simulink model "cell_model_final2"  (R2023a)
settings: Solver=VariableStepAuto  StartTime=0.0  StopTime=T_e  RelTol=1e-3
libraries: neural x50, fl_lib x11, nesl_utility x11, BatteryEstimators x1, ee_lib x1, spspowerguiLib x1
(part 2 of 2)

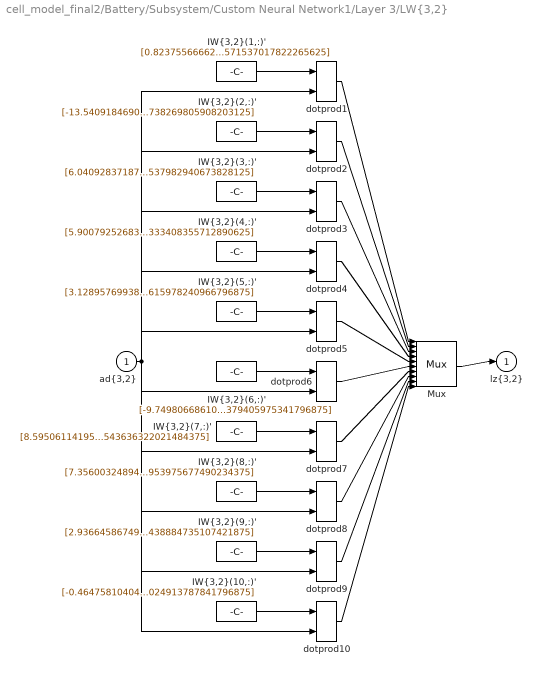
== system cell_model_final2/Battery/Subsystem/Custom Neural Network1/Layer 3/LW{3,2} ==
  "ad{3,2}" : Inport  PortDimensions=10
      mask Display: e = 0.06;c1 = [120 230 180]/255;c2 = ([120 230 180]+0)/(256+128);c3 = ([120 230 180]+128)/(256+128);patch([0 1 1 0],[0 0 1 1],c1);patch([0 1 1 1-e 1-e 0+e],[0 0 1 1-e 0+e 0+e],c2);patch([0 0 1 1-e 0+e 0+e],[0 1 1 1-e 1-e 0+e],c3);plot([0 1 1 0 0],[0 0 1 1 0]);
  "IW{3,2}(1,:)'" : Constant  Value=[0.8237556666211525158161066428874619305133819580078125;0.51571976457906709701006775503628887236118316650390625;-1.72538259025572227045586259919218719005584716796875;5.17857256433064350176209700293838977813720703125;-1.1681412187577204786492757193627767264842987060546875;1.1316882761782769417635563513613305985927581787109375;0.0112615445436738924323005761607419117353856563568115234375;-3.650864637324606309931596115347929298877716064453125;4.0848047341033453250247475807555019855499267578125;-3.444626401094726730889306054450571537017822265625]
      mask Display: e = 0.06;c1 = [120 150 230]/255;c2 = ([120 150 230]+0)/383;c3 = ([120 150 230]+128)/383;patch([0 1 1 0],[0 0 1 1],c1);patch([0 1 1 1-e 1-e 0+e],[0 0 1 1-e 0+e 0+e],c2);patch([0 0 1 1-e 0+e 0+e],[0 1 1 1-e 1-e 0+e],c3);plot([0 1 1 0 0],[0 0 1 1 0]);disp('weights');
  "IW{3,2}(10,:)'" : Constant  Value=[-0.464758104043701714136460623194579966366291046142578125;-0.5992515146409294057860961402184329926967620849609375;-0.251602361335951762999485481486772187054157257080078125;0.6197646560946881155729215606697835028171539306640625;-1.72620687903957392705933671095408499240875244140625;-0.367220886577844185527652598466374911367893218994140625;0.262110630021804624778525294459541328251361846923828125;-16.09438852063943414805180509574711322784423828125;-3.647089595181814303259670850820839405059814453125;-0.442257307555951495459112265962176024913787841796875]
      mask Display: e = 0.06;c1 = [120 150 230]/255;c2 = ([120 150 230]+0)/383;c3 = ([120 150 230]+128)/383;patch([0 1 1 0],[0 0 1 1],c1);patch([0 1 1 1-e 1-e 0+e],[0 0 1 1-e 0+e 0+e],c2);patch([0 0 1 1-e 0+e 0+e],[0 1 1 1-e 1-e 0+e],c3);plot([0 1 1 0 0],[0 0 1 1 0]);disp('weights');
  "IW{3,2}(2,:)'" : Constant  Value=[-13.54091846902824869403048069216310977935791015625;-7.78018168856120784226959585794247686862945556640625;-0.60416965064185490508208431492676027119159698486328125;11.427090964861445598899081232957541942596435546875;-8.1268851032437918746609284426085650920867919921875;2.555711316461996229776332256733439862728118896484375;-6.94223281636129652127920053317211568355560302734375;-3.618245010412151518863765886635519564151763916015625;-2.7533860611985634392340216436423361301422119140625;3.017057444568547186491969114285893738269805908203125]
      mask Display: e = 0.06;c1 = [120 150 230]/255;c2 = ([120 150 230]+0)/383;c3 = ([120 150 230]+128)/383;patch([0 1 1 0],[0 0 1 1],c1);patch([0 1 1 1-e 1-e 0+e],[0 0 1 1-e 0+e 0+e],c2);patch([0 0 1 1-e 0+e 0+e],[0 1 1 1-e 1-e 0+e],c3);plot([0 1 1 0 0],[0 0 1 1 0]);disp('weights');
  "IW{3,2}(3,:)'" : Constant  Value=[6.04092837187769848839025144116021692752838134765625;0.3393572733070511215913711566827259957790374755859375;-0.1361478471900444409126151867894805036485195159912109375;-0.61462706919321596910066318741883151233196258544921875;-1.7451047526482843519346488392329774796962738037109375;-0.8304746157176092768992248238646425306797027587890625;1.5984951728814287275071137628401629626750946044921875;-1.273854906771078265848018418182618916034698486328125;-0.57693518319445968867142937597236596047878265380859375;-1.594857872860516057045288107474334537982940673828125]
      mask Display: e = 0.06;c1 = [120 150 230]/255;c2 = ([120 150 230]+0)/383;c3 = ([120 150 230]+128)/383;patch([0 1 1 0],[0 0 1 1],c1);patch([0 1 1 1-e 1-e 0+e],[0 0 1 1-e 0+e 0+e],c2);patch([0 0 1 1-e 0+e 0+e],[0 1 1 1-e 1-e 0+e],c3);plot([0 1 1 0 0],[0 0 1 1 0]);disp('weights');
  "IW{3,2}(4,:)'" : Constant  Value=[5.9007925268365344351195744820870459079742431640625;-0.65084428298054064487843106689979322254657745361328125;2.17547306835202736152723446139134466648101806640625;-0.97304976004262166977554215918644331395626068115234375;0.23629131647569712182388457222259603440761566162109375;-0.7045430957878242583802830267813988029956817626953125;1.70831633299809926285206529428251087665557861328125;0.2704609371481063728737126439227722585201263427734375;-3.4953864206789848623202487942762672901153564453125;-0.6311199027205882661206715056323446333408355712890625]
      mask Display: e = 0.06;c1 = [120 150 230]/255;c2 = ([120 150 230]+0)/383;c3 = ([120 150 230]+128)/383;patch([0 1 1 0],[0 0 1 1],c1);patch([0 1 1 1-e 1-e 0+e],[0 0 1 1-e 0+e 0+e],c2);patch([0 0 1 1-e 0+e 0+e],[0 1 1 1-e 1-e 0+e],c3);plot([0 1 1 0 0],[0 0 1 1 0]);disp('weights');
  "IW{3,2}(5,:)'" : Constant  Value=[3.128957699389872004758217372000217437744140625;1.075965775142953884113694584812037646770477294921875;0.82378109590055481614712107329978607594966888427734375;-0.6107402140989381944535807633656077086925506591796875;-0.53224852174734793575083813266246579587459564208984375;0.501830234512349537823183709406293928623199462890625;0.11040997298376568902522620874151471070945262908935546875;-0.1498203391362867564762240135678439401090145111083984375;-0.2381298736799780935147197169499122537672519683837890625;-0.653770362514666469877511190134100615978240966796875]
      mask Display: e = 0.06;c1 = [120 150 230]/255;c2 = ([120 150 230]+0)/383;c3 = ([120 150 230]+128)/383;patch([0 1 1 0],[0 0 1 1],c1);patch([0 1 1 1-e 1-e 0+e],[0 0 1 1-e 0+e 0+e],c2);patch([0 0 1 1-e 0+e 0+e],[0 1 1 1-e 1-e 0+e],c3);plot([0 1 1 0 0],[0 0 1 1 0]);disp('weights');
  "IW{3,2}(6,:)'" : Constant  Value=[-9.74980668610820799813154735602438449859619140625;-6.3369232781815441057915450073778629302978515625;6.09327940852977345542740295059047639369964599609375;-4.7027926575543066434192951419390738010406494140625;-5.93152314487222209749006651691161096096038818359375;-15.5812875339934269192099236533977091312408447265625;-0.50925822907497264591114571885555051267147064208984375;2.883830636579010953113311188644729554653167724609375;4.20779319338805724015628584311343729496002197265625;0.10599562508165287499917184277364867739379405975341796875]
      mask Display: e = 0.06;c1 = [120 150 230]/255;c2 = ([120 150 230]+0)/383;c3 = ([120 150 230]+128)/383;patch([0 1 1 0],[0 0 1 1],c1);patch([0 1 1 1-e 1-e 0+e],[0 0 1 1-e 0+e 0+e],c2);patch([0 0 1 1-e 0+e 0+e],[0 1 1 1-e 1-e 0+e],c3);plot([0 1 1 0 0],[0 0 1 1 0]);disp('weights');
  "IW{3,2}(7,:)'" : Constant  Value=[8.5950611419544902247480422374792397022247314453125;1.5635822242984642738150569130084477365016937255859375;3.771727767111268558863912403467111289501190185546875;-1.0919709536841548658259171133977361023426055908203125;11.791071227848863856024763663299381732940673828125;1.6213272379689993574203299431246705353260040283203125;1.5352528648102532482511151101789437234401702880859375;15.361914640598907766388947493396699428558349609375;-11.2104874541272163668281791615299880504608154296875;-19.9152018216922215287922881543636322021484375]
      mask Display: e = 0.06;c1 = [120 150 230]/255;c2 = ([120 150 230]+0)/383;c3 = ([120 150 230]+128)/383;patch([0 1 1 0],[0 0 1 1],c1);patch([0 1 1 1-e 1-e 0+e],[0 0 1 1-e 0+e 0+e],c2);patch([0 0 1 1-e 0+e 0+e],[0 1 1 1-e 1-e 0+e],c3);plot([0 1 1 0 0],[0 0 1 1 0]);disp('weights');
  "IW{3,2}(8,:)'" : Constant  Value=[7.35600324894948442988606984727084636688232421875;0.77271926047475936183417388747329823672771453857421875;0.464109698369803924666854300085105933248996734619140625;0.79881594776103026500635451156995259225368499755859375;-1.193220098882364244019527177442796528339385986328125;-1.7205400623213764621510790675529278814792633056640625;1.884626601101445420027857835520990192890167236328125;-0.85140840144191176630528161695110611617565155029296875;3.348620010332649332696064448100514709949493408203125;0.518919361702509629452606532140634953975677490234375]
      mask Display: e = 0.06;c1 = [120 150 230]/255;c2 = ([120 150 230]+0)/383;c3 = ([120 150 230]+128)/383;patch([0 1 1 0],[0 0 1 1],c1);patch([0 1 1 1-e 1-e 0+e],[0 0 1 1-e 0+e 0+e],c2);patch([0 0 1 1-e 0+e 0+e],[0 1 1 1-e 1-e 0+e],c3);plot([0 1 1 0 0],[0 0 1 1 0]);disp('weights');
  "IW{3,2}(9,:)'" : Constant  Value=[2.9366458674975319809163920581340789794921875;0.11382377123805066665429563954603509046137332916259765625;-0.180298572854895533534858031998737715184688568115234375;-1.4519372197763338316889303314383141696453094482421875;2.490459681232118693827715105726383626461029052734375;-1.0414472033151138674611502210609614849090576171875;-3.008464300367092558730064411065541207790374755859375;1.7983374122680337858781740578706376254558563232421875;-0.14493642436333631362543883369653485715389251708984375;0.08730435018556663429034614409829373471438884735107421875]
      mask Display: e = 0.06;c1 = [120 150 230]/255;c2 = ([120 150 230]+0)/383;c3 = ([120 150 230]+128)/383;patch([0 1 1 0],[0 0 1 1],c1);patch([0 1 1 1-e 1-e 0+e],[0 0 1 1-e 0+e 0+e],c2);patch([0 0 1 1-e 0+e 0+e],[0 1 1 1-e 1-e 0+e],c3);plot([0 1 1 0 0],[0 0 1 1 0]);disp('weights');
  Mux : Mux  Inputs=10
      mask Display: e = 0.06;c1 = [120 150 230]/255;c2 = ([120 150 230]+0)/383;c3 = ([120 150 230]+128)/383;patch([0 1 1 0],[0 0 1 1],c1);patch([0 1 1 1-e 1-e 0+e],[0 0 1 1-e 0+e 0+e],c2);patch([0 0 1 1-e 0+e 0+e],[0 1 1 1-e 1-e 0+e],c3);plot([0 1 1 0 0],[0 0 1 1 0]);disp('Mux');
  dotprod{1..10} (10 alike) : neural/Weight Functions/dotprod
  "lz{3,2}" : Outport
      mask Display: e = 0.06;c1 = [120 230 180]/255;c2 = ([120 230 180]+0)/(256+128);c3 = ([120 230 180]+128)/(256+128);patch([0 1 1 0],[0 0 1 1],c1);patch([0 1 1 1-e 1-e 0+e],[0 0 1 1-e 0+e 0+e],c2);patch([0 0 1 1-e 0+e 0+e],[0 1 1 1-e 1-e 0+e],c3);plot([0 1 1 0 0],[0 0 1 1 0]);
  wires:
  "IW{3,2}(1,:)'"/1 -> dotprod1/1
  "ad{3,2}"/1 -> dotprod1/2, dotprod2/2, dotprod3/2, dotprod4/2, dotprod5/2, dotprod6/2, dotprod7/2, dotprod8/2, dotprod9/2, dotprod10/2
  dotprod1/1 -> Mux/1
  "IW{3,2}(2,:)'"/1 -> dotprod2/1
  dotprod2/1 -> Mux/2
  "IW{3,2}(3,:)'"/1 -> dotprod3/1
  dotprod3/1 -> Mux/3
  "IW{3,2}(4,:)'"/1 -> dotprod4/1
  dotprod4/1 -> Mux/4
  "IW{3,2}(5,:)'"/1 -> dotprod5/1
  dotprod5/1 -> Mux/5
  "IW{3,2}(6,:)'"/1 -> dotprod6/1
  dotprod6/1 -> Mux/6
  "IW{3,2}(7,:)'"/1 -> dotprod7/1
  dotprod7/1 -> Mux/7
  "IW{3,2}(8,:)'"/1 -> dotprod8/1
  dotprod8/1 -> Mux/8
  "IW{3,2}(9,:)'"/1 -> dotprod9/1
  dotprod9/1 -> Mux/9
  "IW{3,2}(10,:)'"/1 -> dotprod10/1
  dotprod10/1 -> Mux/10
  Mux/1 -> "lz{3,2}"/1

== system cell_model_final2/Battery/Subsystem/Custom Neural Network1/Layer 4/Delays 1 ==
  "p{4}" : Inport  PortDimensions=10
      mask Display: e = 0.06;c1 = [120 230 180]/255;c2 = ([120 230 180]+0)/(256+128);c3 = ([120 230 180]+128)/(256+128);patch([0 1 1 0],[0 0 1 1],c1);patch([0 1 1 1-e 1-e 0+e],[0 0 1 1-e 0+e 0+e],c2);patch([0 0 1 1-e 0+e 0+e],[0 1 1 1-e 1-e 0+e],c3);plot([0 1 1 0 0],[0 0 1 1 0]);
  mux : Mux  Inputs=1
      mask Display: e = 0.06;c1 = [120 150 230]/255;c2 = ([120 150 230]+0)/383;c3 = ([120 150 230]+128)/383;patch([0 1 1 0],[0 0 1 1],c1);patch([0 1 1 1-e 1-e 0+e],[0 0 1 1-e 0+e 0+e],c2);patch([0 0 1 1-e 0+e 0+e],[0 1 1 1-e 1-e 0+e],c3);plot([0 1 1 0 0],[0 0 1 1 0]);disp('Mux')
  "pd{4,3}" : Outport
      mask Display: e = 0.06;c1 = [120 230 180]/255;c2 = ([120 230 180]+0)/(256+128);c3 = ([120 230 180]+128)/(256+128);patch([0 1 1 0],[0 0 1 1],c1);patch([0 1 1 1-e 1-e 0+e],[0 0 1 1-e 0+e 0+e],c2);patch([0 0 1 1-e 0+e 0+e],[0 1 1 1-e 1-e 0+e],c3);plot([0 1 1 0 0],[0 0 1 1 0]);
  wires:
  "p{4}"/1 -> mux/1
  mux/1 -> "pd{4,3}"/1

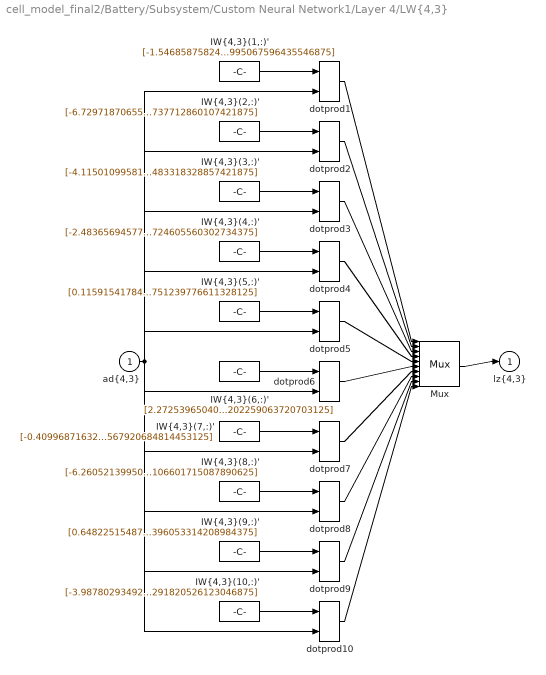
== system cell_model_final2/Battery/Subsystem/Custom Neural Network1/Layer 4/LW{4,3} ==
  "ad{4,3}" : Inport  PortDimensions=10
      mask Display: e = 0.06;c1 = [120 230 180]/255;c2 = ([120 230 180]+0)/(256+128);c3 = ([120 230 180]+128)/(256+128);patch([0 1 1 0],[0 0 1 1],c1);patch([0 1 1 1-e 1-e 0+e],[0 0 1 1-e 0+e 0+e],c2);patch([0 0 1 1-e 0+e 0+e],[0 1 1 1-e 1-e 0+e],c3);plot([0 1 1 0 0],[0 0 1 1 0]);
  "IW{4,3}(1,:)'" : Constant  Value=[-1.546858758243345288718728625099174678325653076171875;-5.41574496058701715384131603059358894824981689453125;-3.346839046542495754721358025562949478626251220703125;0.451767824527080197327677524299360811710357666015625;-6.669883365719584844555356539785861968994140625;-0.62066255443102724687065574471489526331424713134765625;-1.96645724734477322925840780953876674175262451171875;1.31646724517947699695241681183688342571258544921875;-5.08626513682391223625245402217842638492584228515625;0.6517186992629386832476257040980271995067596435546875]
      mask Display: e = 0.06;c1 = [120 150 230]/255;c2 = ([120 150 230]+0)/383;c3 = ([120 150 230]+128)/383;patch([0 1 1 0],[0 0 1 1],c1);patch([0 1 1 1-e 1-e 0+e],[0 0 1 1-e 0+e 0+e],c2);patch([0 0 1 1-e 0+e 0+e],[0 1 1 1-e 1-e 0+e],c3);plot([0 1 1 0 0],[0 0 1 1 0]);disp('weights');
  "IW{4,3}(10,:)'" : Constant  Value=[-3.98780293492059367821411797194741666316986083984375;3.26630480238409592885773236048407852649688720703125;-5.634060446159356416728769545443356037139892578125;1.3065505122799716541948100712033919990062713623046875;4.9805298971298146426534003694541752338409423828125;-6.1388756929773773407532644341699779033660888671875;-0.046357114954881643853479289418828557245433330535888671875;3.15372981633694760006392243667505681514739990234375;7.0811699029023547069527921848930418491363525390625;1.955086813922487731787214215728454291820526123046875]
      mask Display: e = 0.06;c1 = [120 150 230]/255;c2 = ([120 150 230]+0)/383;c3 = ([120 150 230]+128)/383;patch([0 1 1 0],[0 0 1 1],c1);patch([0 1 1 1-e 1-e 0+e],[0 0 1 1-e 0+e 0+e],c2);patch([0 0 1 1-e 0+e 0+e],[0 1 1 1-e 1-e 0+e],c3);plot([0 1 1 0 0],[0 0 1 1 0]);disp('weights');
  "IW{4,3}(2,:)'" : Constant  Value=[-6.72971870655333237465356432949192821979522705078125;1.7518616056329172625538603824679739773273468017578125;9.13726051001393813066897564567625522613525390625;-4.57532989411322699169204497593455016613006591796875;4.633243645744716587842049193568527698516845703125;3.275645115094608872396975129959173500537872314453125;1.1143148869915915355477409320883452892303466796875;-7.5247483965626695834316706168465316295623779296875;17.269833940598214638839635881595313549041748046875;-27.999460156409394784304822678677737712860107421875]
      mask Display: e = 0.06;c1 = [120 150 230]/255;c2 = ([120 150 230]+0)/383;c3 = ([120 150 230]+128)/383;patch([0 1 1 0],[0 0 1 1],c1);patch([0 1 1 1-e 1-e 0+e],[0 0 1 1-e 0+e 0+e],c2);patch([0 0 1 1-e 0+e 0+e],[0 1 1 1-e 1-e 0+e],c3);plot([0 1 1 0 0],[0 0 1 1 0]);disp('weights');
  "IW{4,3}(3,:)'" : Constant  Value=[-4.11501099581523011039507764508016407489776611328125;-0.81767388943092333963846840561018325388431549072265625;1.9110066220211112675286813100683502852916717529296875;-1.0348181098407638334180091987946070730686187744140625;-10.8015348074335815198310228879563510417938232421875;5.81950150578970948345158831216394901275634765625;5.04756186786198046689833063283003866672515869140625;-3.39679740951199082843459109426476061344146728515625;-8.4884899486503844201479296316392719745635986328125;-0.0916084538988721497343448163519497029483318328857421875]
      mask Display: e = 0.06;c1 = [120 150 230]/255;c2 = ([120 150 230]+0)/383;c3 = ([120 150 230]+128)/383;patch([0 1 1 0],[0 0 1 1],c1);patch([0 1 1 1-e 1-e 0+e],[0 0 1 1-e 0+e 0+e],c2);patch([0 0 1 1-e 0+e 0+e],[0 1 1 1-e 1-e 0+e],c3);plot([0 1 1 0 0],[0 0 1 1 0]);disp('weights');
  "IW{4,3}(4,:)'" : Constant  Value=[-2.483656945778097036026110799866728484630584716796875;0.7278102331529456847647452377714216709136962890625;2.740000688501283310216649624635465443134307861328125;-5.623990090066673275259745423682034015655517578125;-0.94208172703027648342555266935960389673709869384765625;1.2687902289863941529546309539000503718852996826171875;2.67200420830051132980997863342054188251495361328125;-2.153123444341618952790895491489209234714508056640625;4.57178011351702284770226469845511019229888916015625;-6.047806784650131106673143221996724605560302734375]
      mask Display: e = 0.06;c1 = [120 150 230]/255;c2 = ([120 150 230]+0)/383;c3 = ([120 150 230]+128)/383;patch([0 1 1 0],[0 0 1 1],c1);patch([0 1 1 1-e 1-e 0+e],[0 0 1 1-e 0+e 0+e],c2);patch([0 0 1 1-e 0+e 0+e],[0 1 1 1-e 1-e 0+e],c3);plot([0 1 1 0 0],[0 0 1 1 0]);disp('weights');
  "IW{4,3}(5,:)'" : Constant  Value=[0.1159154178461006823308565572006045840680599212646484375;-1.8499853959098986333486891453503631055355072021484375;1.2848704877071168706237358492217026650905609130859375;-2.157547822042106933082550312974490225315093994140625;-4.241359906210082186817089677788317203521728515625;0.57736464622362737575400615241960622370243072509765625;-0.01329290190106735027042450525414096773602068424224853515625;-0.74914529347293534744522958135348744690418243408203125;-0.06294257075587723904153136800232459791004657745361328125;-1.23916661798865135324376751668751239776611328125]
      mask Display: e = 0.06;c1 = [120 150 230]/255;c2 = ([120 150 230]+0)/383;c3 = ([120 150 230]+128)/383;patch([0 1 1 0],[0 0 1 1],c1);patch([0 1 1 1-e 1-e 0+e],[0 0 1 1-e 0+e 0+e],c2);patch([0 0 1 1-e 0+e 0+e],[0 1 1 1-e 1-e 0+e],c3);plot([0 1 1 0 0],[0 0 1 1 0]);disp('weights');
  "IW{4,3}(6,:)'" : Constant  Value=[2.2725396504043171574949155910871922969818115234375;1.73565961087123010742061524069868028163909912109375;-1.569911766278661247042691684328019618988037109375;3.30693627073573903629721826291643083095550537109375;0.05289787163614211029649680995134986005723476409912109375;-8.7957836952562242771591627388261258602142333984375;2.29184513753000640434720480698160827159881591796875;-2.832488029926452099971356801688671112060546875;0.7825427923264813845349863186129368841648101806640625;-3.85471441436257311607960218680091202259063720703125]
      mask Display: e = 0.06;c1 = [120 150 230]/255;c2 = ([120 150 230]+0)/383;c3 = ([120 150 230]+128)/383;patch([0 1 1 0],[0 0 1 1],c1);patch([0 1 1 1-e 1-e 0+e],[0 0 1 1-e 0+e 0+e],c2);patch([0 0 1 1-e 0+e 0+e],[0 1 1 1-e 1-e 0+e],c3);plot([0 1 1 0 0],[0 0 1 1 0]);disp('weights');
  "IW{4,3}(7,:)'" : Constant  Value=[-0.409968716321139903246972835404449142515659332275390625;-0.6642236348449463978482754100696183741092681884765625;2.4107726960936570748117446782998740673065185546875;3.3503577009520579821355568128637969493865966796875;-3.37791576775854185399339257855899631977081298828125;-4.03534815408382296908484931918792426586151123046875;0.88018778310807543885374570891144685447216033935546875;3.60491302059822782410947183961980044841766357421875;5.2728163588108483139649251825176179409027099609375;0.171802163157868836851349669814226217567920684814453125]
      mask Display: e = 0.06;c1 = [120 150 230]/255;c2 = ([120 150 230]+0)/383;c3 = ([120 150 230]+128)/383;patch([0 1 1 0],[0 0 1 1],c1);patch([0 1 1 1-e 1-e 0+e],[0 0 1 1-e 0+e 0+e],c2);patch([0 0 1 1-e 0+e 0+e],[0 1 1 1-e 1-e 0+e],c3);plot([0 1 1 0 0],[0 0 1 1 0]);disp('weights');
  "IW{4,3}(8,:)'" : Constant  Value=[-6.26052139950341679508483139215968549251556396484375;14.977608629465382961143404827453196048736572265625;-12.272214380771313102513886406086385250091552734375;13.1246927787515037522325656027533113956451416015625;-3.196246741237889654740911282715387642383575439453125;4.721382732960687889089967939071357250213623046875;0.90901296199383907481461619681795127689838409423828125;-4.89929433066750785741305662668310105800628662109375;14.120534296999966983321428415365517139434814453125;10.1202950796688586621030481182970106601715087890625]
      mask Display: e = 0.06;c1 = [120 150 230]/255;c2 = ([120 150 230]+0)/383;c3 = ([120 150 230]+128)/383;patch([0 1 1 0],[0 0 1 1],c1);patch([0 1 1 1-e 1-e 0+e],[0 0 1 1-e 0+e 0+e],c2);patch([0 0 1 1-e 0+e 0+e],[0 1 1 1-e 1-e 0+e],c3);plot([0 1 1 0 0],[0 0 1 1 0]);disp('weights');
  "IW{4,3}(9,:)'" : Constant  Value=[0.648225154879653597816968613187782466411590576171875;14.361668336610517116014307248406112194061279296875;2.986517236766482508159015196724794805049896240234375;-8.499556907750882572827322292141616344451904296875;14.8883666792993221150709359790198504924774169921875;11.4168531391206879987976208212785422801971435546875;-10.8986631467053118882404305622912943363189697265625;-15.0582136542635165454839807352982461452484130859375;-0.86265019356548078288682290803990326821804046630859375;-24.31247704679903876012758701108396053314208984375]
      mask Display: e = 0.06;c1 = [120 150 230]/255;c2 = ([120 150 230]+0)/383;c3 = ([120 150 230]+128)/383;patch([0 1 1 0],[0 0 1 1],c1);patch([0 1 1 1-e 1-e 0+e],[0 0 1 1-e 0+e 0+e],c2);patch([0 0 1 1-e 0+e 0+e],[0 1 1 1-e 1-e 0+e],c3);plot([0 1 1 0 0],[0 0 1 1 0]);disp('weights');
  Mux : Mux  Inputs=10
      mask Display: e = 0.06;c1 = [120 150 230]/255;c2 = ([120 150 230]+0)/383;c3 = ([120 150 230]+128)/383;patch([0 1 1 0],[0 0 1 1],c1);patch([0 1 1 1-e 1-e 0+e],[0 0 1 1-e 0+e 0+e],c2);patch([0 0 1 1-e 0+e 0+e],[0 1 1 1-e 1-e 0+e],c3);plot([0 1 1 0 0],[0 0 1 1 0]);disp('Mux');
  dotprod{1..10} (10 alike) : neural/Weight Functions/dotprod
  "lz{4,3}" : Outport
      mask Display: e = 0.06;c1 = [120 230 180]/255;c2 = ([120 230 180]+0)/(256+128);c3 = ([120 230 180]+128)/(256+128);patch([0 1 1 0],[0 0 1 1],c1);patch([0 1 1 1-e 1-e 0+e],[0 0 1 1-e 0+e 0+e],c2);patch([0 0 1 1-e 0+e 0+e],[0 1 1 1-e 1-e 0+e],c3);plot([0 1 1 0 0],[0 0 1 1 0]);
  wires:
  "IW{4,3}(1,:)'"/1 -> dotprod1/1
  "ad{4,3}"/1 -> dotprod1/2, dotprod2/2, dotprod3/2, dotprod4/2, dotprod5/2, dotprod6/2, dotprod7/2, dotprod8/2, dotprod9/2, dotprod10/2
  dotprod1/1 -> Mux/1
  "IW{4,3}(2,:)'"/1 -> dotprod2/1
  dotprod2/1 -> Mux/2
  "IW{4,3}(3,:)'"/1 -> dotprod3/1
  dotprod3/1 -> Mux/3
  "IW{4,3}(4,:)'"/1 -> dotprod4/1
  dotprod4/1 -> Mux/4
  "IW{4,3}(5,:)'"/1 -> dotprod5/1
  dotprod5/1 -> Mux/5
  "IW{4,3}(6,:)'"/1 -> dotprod6/1
  dotprod6/1 -> Mux/6
  "IW{4,3}(7,:)'"/1 -> dotprod7/1
  dotprod7/1 -> Mux/7
  "IW{4,3}(8,:)'"/1 -> dotprod8/1
  dotprod8/1 -> Mux/8
  "IW{4,3}(9,:)'"/1 -> dotprod9/1
  dotprod9/1 -> Mux/9
  "IW{4,3}(10,:)'"/1 -> dotprod10/1
  dotprod10/1 -> Mux/10
  Mux/1 -> "lz{4,3}"/1

== system cell_model_final2/Battery/Subsystem/Custom Neural Network1/Layer 5/Delays 1 ==
  "p{5}" : Inport  PortDimensions=10
      mask Display: e = 0.06;c1 = [120 230 180]/255;c2 = ([120 230 180]+0)/(256+128);c3 = ([120 230 180]+128)/(256+128);patch([0 1 1 0],[0 0 1 1],c1);patch([0 1 1 1-e 1-e 0+e],[0 0 1 1-e 0+e 0+e],c2);patch([0 0 1 1-e 0+e 0+e],[0 1 1 1-e 1-e 0+e],c3);plot([0 1 1 0 0],[0 0 1 1 0]);
  mux : Mux  Inputs=1
      mask Display: e = 0.06;c1 = [120 150 230]/255;c2 = ([120 150 230]+0)/383;c3 = ([120 150 230]+128)/383;patch([0 1 1 0],[0 0 1 1],c1);patch([0 1 1 1-e 1-e 0+e],[0 0 1 1-e 0+e 0+e],c2);patch([0 0 1 1-e 0+e 0+e],[0 1 1 1-e 1-e 0+e],c3);plot([0 1 1 0 0],[0 0 1 1 0]);disp('Mux')
  "pd{5,4}" : Outport
      mask Display: e = 0.06;c1 = [120 230 180]/255;c2 = ([120 230 180]+0)/(256+128);c3 = ([120 230 180]+128)/(256+128);patch([0 1 1 0],[0 0 1 1],c1);patch([0 1 1 1-e 1-e 0+e],[0 0 1 1-e 0+e 0+e],c2);patch([0 0 1 1-e 0+e 0+e],[0 1 1 1-e 1-e 0+e],c3);plot([0 1 1 0 0],[0 0 1 1 0]);
  wires:
  "p{5}"/1 -> mux/1
  mux/1 -> "pd{5,4}"/1

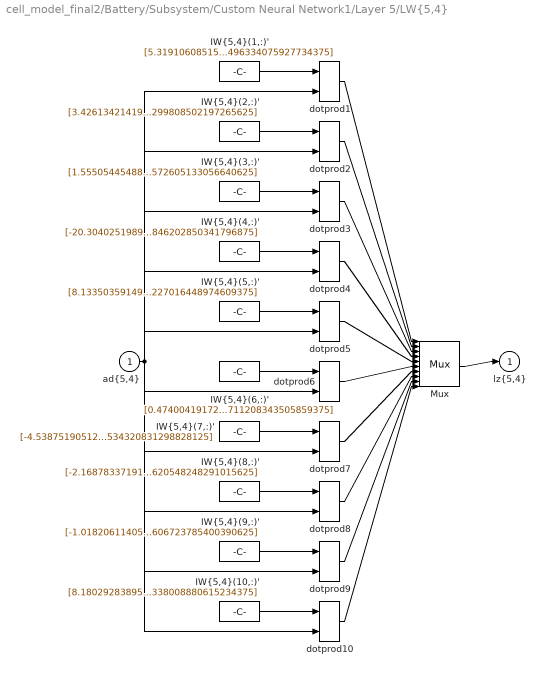
== system cell_model_final2/Battery/Subsystem/Custom Neural Network1/Layer 5/LW{5,4} ==
  "ad{5,4}" : Inport  PortDimensions=10
      mask Display: e = 0.06;c1 = [120 230 180]/255;c2 = ([120 230 180]+0)/(256+128);c3 = ([120 230 180]+128)/(256+128);patch([0 1 1 0],[0 0 1 1],c1);patch([0 1 1 1-e 1-e 0+e],[0 0 1 1-e 0+e 0+e],c2);patch([0 0 1 1-e 0+e 0+e],[0 1 1 1-e 1-e 0+e],c3);plot([0 1 1 0 0],[0 0 1 1 0]);
  "IW{5,4}(1,:)'" : Constant  Value=[5.31910608515874283597213434404693543910980224609375;-37.6187219247760680218561901710927486419677734375;-1.434327602098746989867095180670730769634246826171875;-1.3067931540625294939417244677315466105937957763671875;0.08338336636821926106666325040350784547626972198486328125;3.10444042714829127049824819550849497318267822265625;3.20260944459612328927278213086538016796112060546875;0.69515320195009311365907933577545918524265289306640625;1.22868083139611439236205114866606891155242919921875;-5.956084539158521096169351949356496334075927734375]
      mask Display: e = 0.06;c1 = [120 150 230]/255;c2 = ([120 150 230]+0)/383;c3 = ([120 150 230]+128)/383;patch([0 1 1 0],[0 0 1 1],c1);patch([0 1 1 1-e 1-e 0+e],[0 0 1 1-e 0+e 0+e],c2);patch([0 0 1 1-e 0+e 0+e],[0 1 1 1-e 1-e 0+e],c3);plot([0 1 1 0 0],[0 0 1 1 0]);disp('weights');
  "IW{5,4}(10,:)'" : Constant  Value=[8.18029283895581471597324707545340061187744140625;-0.86604032375827444401039656440843828022480010986328125;10.406226965972205533716987702064216136932373046875;-8.485710592220481629510686616413295269012451171875;-0.251726104378499015989945064575294964015483856201171875;20.0634977846928421740813064388930797576904296875;-1.366718568608316086709919545683078467845916748046875;27.82724288856896777133442810736596584320068359375;4.8484804648080181976865787873975932598114013671875;3.57714877656545038320246021612547338008880615234375]
      mask Display: e = 0.06;c1 = [120 150 230]/255;c2 = ([120 150 230]+0)/383;c3 = ([120 150 230]+128)/383;patch([0 1 1 0],[0 0 1 1],c1);patch([0 1 1 1-e 1-e 0+e],[0 0 1 1-e 0+e 0+e],c2);patch([0 0 1 1-e 0+e 0+e],[0 1 1 1-e 1-e 0+e],c3);plot([0 1 1 0 0],[0 0 1 1 0]);disp('weights');
  "IW{5,4}(2,:)'" : Constant  Value=[3.42613421419545005619511357508599758148193359375;1.114618823772122624404801172204315662384033203125;-6.75680619223893419444948449381627142429351806640625;-1.91855581646149797592215691111050546169281005859375;-3.572382975305118169018214757670648396015167236328125;4.45780515936019838818538119085133075714111328125;-5.79158021666007538641451901639811694622039794921875;4.38311052670753742432907529291696846485137939453125;-1.7471431694872290307785078766755759716033935546875;-1.199354747415134259114211090491153299808502197265625]
      mask Display: e = 0.06;c1 = [120 150 230]/255;c2 = ([120 150 230]+0)/383;c3 = ([120 150 230]+128)/383;patch([0 1 1 0],[0 0 1 1],c1);patch([0 1 1 1-e 1-e 0+e],[0 0 1 1-e 0+e 0+e],c2);patch([0 0 1 1-e 0+e 0+e],[0 1 1 1-e 1-e 0+e],c3);plot([0 1 1 0 0],[0 0 1 1 0]);disp('weights');
  "IW{5,4}(3,:)'" : Constant  Value=[1.555054454884164716332861644332297146320343017578125;0.280436030021297078018704951318795792758464813232421875;-1.340061650945262083922671081381849944591522216796875;1.6251508867869788321769419781048782169818878173828125;-1.0157386511680421836700816129450686275959014892578125;-5.35130459212175946248635227675549685955047607421875;0.76519595505605464413889649222255684435367584228515625;0.2585494067780447213777961223968304693698883056640625;0.7317476832289095955985658292775042355060577392578125;-1.637176688866903706554012387641705572605133056640625]
      mask Display: e = 0.06;c1 = [120 150 230]/255;c2 = ([120 150 230]+0)/383;c3 = ([120 150 230]+128)/383;patch([0 1 1 0],[0 0 1 1],c1);patch([0 1 1 1-e 1-e 0+e],[0 0 1 1-e 0+e 0+e],c2);patch([0 0 1 1-e 0+e 0+e],[0 1 1 1-e 1-e 0+e],c3);plot([0 1 1 0 0],[0 0 1 1 0]);disp('weights');
  "IW{5,4}(4,:)'" : Constant  Value=[-20.30402519890122903234441764652729034423828125;22.457629621246137929801989230327308177947998046875;0.314878492933852116575366153483628295361995697021484375;-44.36293643056806246249834657646715641021728515625;7.3827011574238969870975779485888779163360595703125;-35.88281999329792171238295850344002246856689453125;60.188644212525076682140934281051158905029296875;-8.9725237313902770353024607175029814243316650390625;-7.32605500412379928576456222799606621265411376953125;20.154382584722309701419362681917846202850341796875]
      mask Display: e = 0.06;c1 = [120 150 230]/255;c2 = ([120 150 230]+0)/383;c3 = ([120 150 230]+128)/383;patch([0 1 1 0],[0 0 1 1],c1);patch([0 1 1 1-e 1-e 0+e],[0 0 1 1-e 0+e 0+e],c2);patch([0 0 1 1-e 0+e 0+e],[0 1 1 1-e 1-e 0+e],c3);plot([0 1 1 0 0],[0 0 1 1 0]);disp('weights');
  "IW{5,4}(5,:)'" : Constant  Value=[8.1335035914949518343064482905901968479156494140625;15.49384820678261576176737435162067413330078125;37.736545982073863569894456304609775543212890625;-13.3628093022243650267455450375564396381378173828125;-8.62393036572091631342118489556014537811279296875;-16.40819498321757663461539777927100658416748046875;-3.410303327601974299199127926840446889400482177734375;24.133962885927786601314437575638294219970703125;-16.080026613818450442749963258393108844757080078125;9.37803262099551915298434323631227016448974609375]
      mask Display: e = 0.06;c1 = [120 150 230]/255;c2 = ([120 150 230]+0)/383;c3 = ([120 150 230]+128)/383;patch([0 1 1 0],[0 0 1 1],c1);patch([0 1 1 1-e 1-e 0+e],[0 0 1 1-e 0+e 0+e],c2);patch([0 0 1 1-e 0+e 0+e],[0 1 1 1-e 1-e 0+e],c3);plot([0 1 1 0 0],[0 0 1 1 0]);disp('weights');
  "IW{5,4}(6,:)'" : Constant  Value=[0.474004191724247625483457113659824244678020477294921875;-0.771879334027128383155513802194036543369293212890625;1.25980116172532152774010683060623705387115478515625;5.09481225898411604902094040880911052227020263671875;-6.057666156447250926930792047642171382904052734375;1.0032813129573601163002649627742357552051544189453125;0.54980960210650720032532490222365595400333404541015625;5.677288355257385177310425206087529659271240234375;3.371131008149129026918444651528261601924896240234375;0.339900525159732236346599165699444711208343505859375]
      mask Display: e = 0.06;c1 = [120 150 230]/255;c2 = ([120 150 230]+0)/383;c3 = ([120 150 230]+128)/383;patch([0 1 1 0],[0 0 1 1],c1);patch([0 1 1 1-e 1-e 0+e],[0 0 1 1-e 0+e 0+e],c2);patch([0 0 1 1-e 0+e 0+e],[0 1 1 1-e 1-e 0+e],c3);plot([0 1 1 0 0],[0 0 1 1 0]);disp('weights');
  "IW{5,4}(7,:)'" : Constant  Value=[-4.53875190512472048709469163441099226474761962890625;-1.27624362940507030117487374809570610523223876953125;-0.5325326436101438520864803649601526558399200439453125;-0.76454466657364406056984762471984140574932098388671875;1.3293898148616258847454218994244001805782318115234375;8.2016192404383243541587944491766393184661865234375;-0.420980338568227863138559996514231897890567779541015625;-0.32581960761651063140931228190311230719089508056640625;3.68923545619525139471761576714925467967987060546875;3.654730298709310876148492752690799534320831298828125]
      mask Display: e = 0.06;c1 = [120 150 230]/255;c2 = ([120 150 230]+0)/383;c3 = ([120 150 230]+128)/383;patch([0 1 1 0],[0 0 1 1],c1);patch([0 1 1 1-e 1-e 0+e],[0 0 1 1-e 0+e 0+e],c2);patch([0 0 1 1-e 0+e 0+e],[0 1 1 1-e 1-e 0+e],c3);plot([0 1 1 0 0],[0 0 1 1 0]);disp('weights');
  "IW{5,4}(8,:)'" : Constant  Value=[-2.1687833719175610980300916708074510097503662109375;-1.555262101477545844119276807759888470172882080078125;3.63732074692894880030280546634458005428314208984375;-2.926721780427193220219805880333296954631805419921875;-3.199812050957930420480579414288513362407684326171875;3.306279673153628362314293553936295211315155029296875;-1.710894450984811410165775669156573712825775146484375;-0.958158604621420550984112196601927280426025390625;1.156343479755686853849283579620532691478729248046875;6.4019059577235708502485067583620548248291015625]
      mask Display: e = 0.06;c1 = [120 150 230]/255;c2 = ([120 150 230]+0)/383;c3 = ([120 150 230]+128)/383;patch([0 1 1 0],[0 0 1 1],c1);patch([0 1 1 1-e 1-e 0+e],[0 0 1 1-e 0+e 0+e],c2);patch([0 0 1 1-e 0+e 0+e],[0 1 1 1-e 1-e 0+e],c3);plot([0 1 1 0 0],[0 0 1 1 0]);disp('weights');
  "IW{5,4}(9,:)'" : Constant  Value=[-1.018206114054226230081212634104304015636444091796875;0.049203477607104494084833135048029362224042415618896484375;1.100856722356188921452258000499568879604339599609375;-0.048629482677228268172608949271307210437953472137451171875;-0.353114170971075946869888184664887376129627227783203125;-0.09062537123318527287896273492151522077620029449462890625;-0.77821592155081731334576033987104892730712890625;-0.208814446511384643745401490377844311296939849853515625;-0.6086582230673425186751046567223966121673583984375;1.30310740687895876277480056160129606723785400390625]
      mask Display: e = 0.06;c1 = [120 150 230]/255;c2 = ([120 150 230]+0)/383;c3 = ([120 150 230]+128)/383;patch([0 1 1 0],[0 0 1 1],c1);patch([0 1 1 1-e 1-e 0+e],[0 0 1 1-e 0+e 0+e],c2);patch([0 0 1 1-e 0+e 0+e],[0 1 1 1-e 1-e 0+e],c3);plot([0 1 1 0 0],[0 0 1 1 0]);disp('weights');
  Mux : Mux  Inputs=10
      mask Display: e = 0.06;c1 = [120 150 230]/255;c2 = ([120 150 230]+0)/383;c3 = ([120 150 230]+128)/383;patch([0 1 1 0],[0 0 1 1],c1);patch([0 1 1 1-e 1-e 0+e],[0 0 1 1-e 0+e 0+e],c2);patch([0 0 1 1-e 0+e 0+e],[0 1 1 1-e 1-e 0+e],c3);plot([0 1 1 0 0],[0 0 1 1 0]);disp('Mux');
  dotprod{1..10} (10 alike) : neural/Weight Functions/dotprod
  "lz{5,4}" : Outport
      mask Display: e = 0.06;c1 = [120 230 180]/255;c2 = ([120 230 180]+0)/(256+128);c3 = ([120 230 180]+128)/(256+128);patch([0 1 1 0],[0 0 1 1],c1);patch([0 1 1 1-e 1-e 0+e],[0 0 1 1-e 0+e 0+e],c2);patch([0 0 1 1-e 0+e 0+e],[0 1 1 1-e 1-e 0+e],c3);plot([0 1 1 0 0],[0 0 1 1 0]);
  wires:
  "IW{5,4}(1,:)'"/1 -> dotprod1/1
  "ad{5,4}"/1 -> dotprod1/2, dotprod2/2, dotprod3/2, dotprod4/2, dotprod5/2, dotprod6/2, dotprod7/2, dotprod8/2, dotprod9/2, dotprod10/2
  dotprod1/1 -> Mux/1
  "IW{5,4}(2,:)'"/1 -> dotprod2/1
  dotprod2/1 -> Mux/2
  "IW{5,4}(3,:)'"/1 -> dotprod3/1
  dotprod3/1 -> Mux/3
  "IW{5,4}(4,:)'"/1 -> dotprod4/1
  dotprod4/1 -> Mux/4
  "IW{5,4}(5,:)'"/1 -> dotprod5/1
  dotprod5/1 -> Mux/5
  "IW{5,4}(6,:)'"/1 -> dotprod6/1
  dotprod6/1 -> Mux/6
  "IW{5,4}(7,:)'"/1 -> dotprod7/1
  dotprod7/1 -> Mux/7
  "IW{5,4}(8,:)'"/1 -> dotprod8/1
  dotprod8/1 -> Mux/8
  "IW{5,4}(9,:)'"/1 -> dotprod9/1
  dotprod9/1 -> Mux/9
  "IW{5,4}(10,:)'"/1 -> dotprod10/1
  dotprod10/1 -> Mux/10
  Mux/1 -> "lz{5,4}"/1

== system cell_model_final2/Battery/Subsystem/Custom Neural Network1/Layer 6/Delays 1 ==
  "p{6}" : Inport  PortDimensions=10
      mask Display: e = 0.06;c1 = [120 230 180]/255;c2 = ([120 230 180]+0)/(256+128);c3 = ([120 230 180]+128)/(256+128);patch([0 1 1 0],[0 0 1 1],c1);patch([0 1 1 1-e 1-e 0+e],[0 0 1 1-e 0+e 0+e],c2);patch([0 0 1 1-e 0+e 0+e],[0 1 1 1-e 1-e 0+e],c3);plot([0 1 1 0 0],[0 0 1 1 0]);
  mux : Mux  Inputs=1
      mask Display: e = 0.06;c1 = [120 150 230]/255;c2 = ([120 150 230]+0)/383;c3 = ([120 150 230]+128)/383;patch([0 1 1 0],[0 0 1 1],c1);patch([0 1 1 1-e 1-e 0+e],[0 0 1 1-e 0+e 0+e],c2);patch([0 0 1 1-e 0+e 0+e],[0 1 1 1-e 1-e 0+e],c3);plot([0 1 1 0 0],[0 0 1 1 0]);disp('Mux')
  "pd{6,5}" : Outport
      mask Display: e = 0.06;c1 = [120 230 180]/255;c2 = ([120 230 180]+0)/(256+128);c3 = ([120 230 180]+128)/(256+128);patch([0 1 1 0],[0 0 1 1],c1);patch([0 1 1 1-e 1-e 0+e],[0 0 1 1-e 0+e 0+e],c2);patch([0 0 1 1-e 0+e 0+e],[0 1 1 1-e 1-e 0+e],c3);plot([0 1 1 0 0],[0 0 1 1 0]);
  wires:
  "p{6}"/1 -> mux/1
  mux/1 -> "pd{6,5}"/1

== system cell_model_final2/Battery/Subsystem/Custom Neural Network1/Layer 6/LW{6,5} ==
  "ad{6,5}" : Inport  PortDimensions=10
      mask Display: e = 0.06;c1 = [120 230 180]/255;c2 = ([120 230 180]+0)/(256+128);c3 = ([120 230 180]+128)/(256+128);patch([0 1 1 0],[0 0 1 1],c1);patch([0 1 1 1-e 1-e 0+e],[0 0 1 1-e 0+e 0+e],c2);patch([0 0 1 1-e 0+e 0+e],[0 1 1 1-e 1-e 0+e],c3);plot([0 1 1 0 0],[0 0 1 1 0]);
  "IW{6,5}(1,:)'" : Constant  Value=[-0.406429640109170875472699435704271309077739715576171875;-0.267371167482458316211335613843402825295925140380859375;-0.71984747692384021267031357638188637793064117431640625;0.043158778961537129503778231764954398386180400848388671875;0.04783387904272039248265713240471086464822292327880859375;0.2008960714624491716850940292715677060186862945556640625;-0.40349557711881012256327494469587691128253936767578125;-0.2021370367535566814343184205426950938999652862548828125;-1.0259539320283483920803746514138765633106231689453125;-0.09320849323068969294325825103442184627056121826171875]
      mask Display: e = 0.06;c1 = [120 150 230]/255;c2 = ([120 150 230]+0)/383;c3 = ([120 150 230]+128)/383;patch([0 1 1 0],[0 0 1 1],c1);patch([0 1 1 1-e 1-e 0+e],[0 0 1 1-e 0+e 0+e],c2);patch([0 0 1 1-e 0+e 0+e],[0 1 1 1-e 1-e 0+e],c3);plot([0 1 1 0 0],[0 0 1 1 0]);disp('weights');
  Mux : Mux  Inputs=1
      mask Display: e = 0.06;c1 = [120 150 230]/255;c2 = ([120 150 230]+0)/383;c3 = ([120 150 230]+128)/383;patch([0 1 1 0],[0 0 1 1],c1);patch([0 1 1 1-e 1-e 0+e],[0 0 1 1-e 0+e 0+e],c2);patch([0 0 1 1-e 0+e 0+e],[0 1 1 1-e 1-e 0+e],c3);plot([0 1 1 0 0],[0 0 1 1 0]);disp('Mux');
  dotprod1 : neural/Weight Functions/dotprod
  "lz{6,5}" : Outport
      mask Display: e = 0.06;c1 = [120 230 180]/255;c2 = ([120 230 180]+0)/(256+128);c3 = ([120 230 180]+128)/(256+128);patch([0 1 1 0],[0 0 1 1],c1);patch([0 1 1 1-e 1-e 0+e],[0 0 1 1-e 0+e 0+e],c2);patch([0 0 1 1-e 0+e 0+e],[0 1 1 1-e 1-e 0+e],c3);plot([0 1 1 0 0],[0 0 1 1 0]);
  wires:
  "IW{6,5}(1,:)'"/1 -> dotprod1/1
  "ad{6,5}"/1 -> dotprod1/2
  dotprod1/1 -> Mux/1
  Mux/1 -> "lz{6,5}"/1

== matlab function cell_model_final2/Battery/Subsystem/MATLAB Function ==
  data: u input; y output; v input; w input
function y = fcn(u,v,w)


all=[u;v;w];

y = all;
